simulink model "drive1m_real"  (R2022a)
settings: Solver=FixedStepAuto  StartTime=0.0  StopTime=10.0  RelTol=1e-3  EnableMultiTasking=on
values from neighbouring files (symbols this model uses):
  ticksPerRot = 20    [robotParameters.m]
  wheelR = 0.031    [robotParameters.m]
undefined symbols (not defined in the file or in its folder): InputPWM, WheelSpeed
libraries: arduinolib x8, slpidlib x1, mobileRoboticsTrainingLib x1
settings Model: ExtModeTrigDuration=2  Creator=heath  LastModifiedBy=heath
settings OptimizationCC: EnhancedBackFolding=on  PassReuseOutputArgsAs=Individual arguments  ZeroExternalMemoryAtStartup=off  ZeroInternalMemoryAtStartup=off  MaxStackSize=64  OptimizeBlockOrder=speed  DifferentSizesBufferReuse=on  OptimizationCustomize=off  EfficientTunableParamExpr=on
settings DebuggingCC: ParameterTunabilityLossMsg=error
settings HardwareCC: ProdBitPerPointer=32  ProdBitPerSizeT=32  ProdBitPerPtrDiffT=32  ProdLargestAtomicInteger=Long  ProdLargestAtomicFloat=Double  ProdWordSize=32  ProdHWDeviceType=ARM Compatible->ARM Cortex  UseEmbeddedCoderFeatures=off  UseSimulinkCoderFeatures=off
settings SFSimCC: MATLABDynamicMemAlloc=off
settings RTWCC: SystemTargetFile=ert.tlc  HardwareBoard=Arduino Nano 33 IoT  TemplateMakefile=ert_default_tmf  Toolchain=Arduino ARM  BuildConfiguration=Faster Runs
settings CodeAppCC: ForceParamTrailComments=on  IgnoreCustomStorageClasses=off  OperatorAnnotations=on  SimulinkDataObjDesc=on  SFDataObjDesc=on  InsertBlockDesc=on
settings ERTTargetCC: SupportContinuousTime=on  SupportNonInlinedSFcns=on  SupportVariableSizeSignals=on  ExtModeTransport=3  ExtModeStaticAlloc=on  ExtModeStaticAllocSize=8192  ExtModeMexFile=ext_xcp  ExtModeIntrfLevel=Level2 - Open

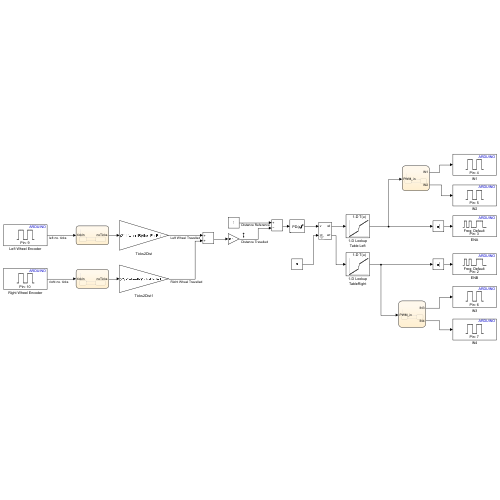
[thumbnail: Simulink's stored preview of the top-level diagram]
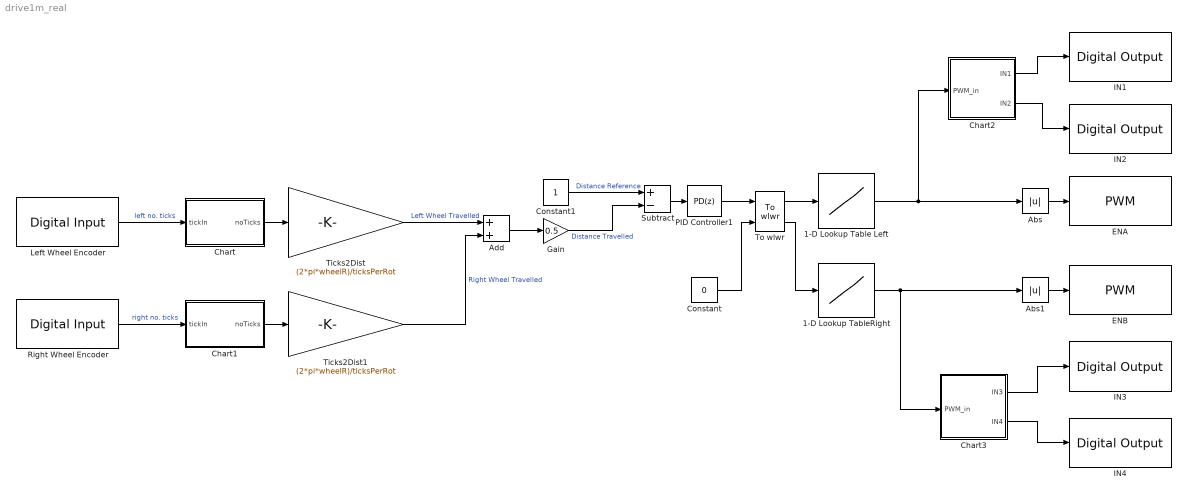
== system drive1m_real ==
  1-D Lookup Table Left : Lookup_n-D  NumberOfTableDimensions=1  BreakpointsForDimension1=WheelSpeed  Table=InputPWM  InternalRulePriority=Speed  RndMeth=Simplest
  1-D Lookup TableRight : Lookup_n-D  NumberOfTableDimensions=1  BreakpointsForDimension1=WheelSpeed  Table=InputPWM  InternalRulePriority=Speed  RndMeth=Simplest
  Abs : Abs  SaturateOnIntegerOverflow=off
  Abs1 : Abs  SaturateOnIntegerOverflow=off
  Add : Sum
  Chart : Stateflow chart  TreatAsAtomicUnit=on
  Chart1 : Stateflow chart  TreatAsAtomicUnit=on
  Chart2 : Stateflow chart  TreatAsAtomicUnit=on
  Chart3 : Stateflow chart  TreatAsAtomicUnit=on
  Constant : Constant  Value=0
  Constant1 : Constant
  ENA : arduinolib/PWM  pinNumber=3  frequencyType=Default  desiredFrequency=490.2  achievableFrequency=490.2
  ENB : arduinolib/PWM  pinNumber=2  frequencyType=Default  desiredFrequency=490.2  achievableFrequency=490.2
  Gain : Gain  Gain=0.5
  IN1 : arduinolib/Digital Output  pinNumber=4  Direction=output  blockPlatform=arduino
  IN2 : arduinolib/Digital Output  pinNumber=5  Direction=output  blockPlatform=arduino
  IN3 : arduinolib/Digital Output  pinNumber=6  Direction=output  blockPlatform=arduino
  IN4 : arduinolib/Digital Output  pinNumber=7  Direction=output  blockPlatform=arduino
  Left Wheel Encoder : arduinolib/Digital Input  pinNumber=9  mode=Default  Direction=input  SampleTime=0.1  blockPlatform=arduino
  PID Controller1 : slpidlib/PID Controller  Controller=PD  Form=Parallel  TimeDomain=Discrete-time  UseExternalTs=off  SampleTime=-1  IntegratorMethod=Forward Euler  FilterMethod=Forward Euler  ControllerParametersSource=internal  P=0.856187400165564  I=-30.3503190798584  UseKiTs=off  D=0.221941519902306  N=26.0006664672571  UseFilter=on  TunerSelectOption=Transfer Function Based (PID Tuner App)  InitialConditionSource=internal  InitialConditionForIntegrator=0  InitialConditionForFilter=0  DifferentiatorICPrevScaledInput=0  ExternalReset=none  TrackingMode=off  Kt=1  LimitOutput=on  SatLimitsSource=internal  UpperSaturationLimit=0.5  LowerSaturationLimit=-0.5  LinearizeAsGain=on  AntiWindupMode=clamping  Kb=1  POutMin=[]  POutMax=[]  IOutMin=[]  IOutMax=[]  DOutMin=[]  DOutMax=[]  NOutMin=[]  NOutMax=[]  SumOutMin=[]  SumOutMax=[]  SaturationOutMin=[]  SaturationOutMax=[]  PParamMin=[]  PParamMax=[]  IParamMin=[]  IParamMax=[]  DParamMin=[]  DParamMax=[]  NParamMin=[]  NParamMax=[]  KbParamMin=[]  KbParamMax=[]  KtParamMin=[]  KtParamMax=[]  KbOutMin=[]  KbOutMax=[]  KtOutMin=[]  KtOutMax=[]  IntegratorOutMin=[]  IntegratorOutMax=[]  FilterOutMin=[]  FilterOutMax=[]  SumI1OutMin=[]  SumI1OutMax=[]  SumI2OutMin=[]  SumI2OutMax=[]  SumI3OutMin=[]  SumI3OutMax=[]  SumI4OutMin=[]  SumI4OutMax=[]  SumDOutMin=[]  SumDOutMax=[]  DifferentiatorOutMin=[]  DifferentiatorOutMax=[]  FilterDiffOutCoefMin=[]  FilterDiffOutCoefMax=[]  ReciprocalOutMin=[]  ReciprocalOutMax=[]  SumDenOutMin=[]  SumDenOutMax=[]  SumNumOutMin=[]  SumNumOutMax=[]  DivideOutMin=[]  DivideOutMax=[]  UdiffTsProdOutMin=[]  UdiffTsProdOutMax=[]  NTsProdOutMin=[]  NTsProdOutMax=[]  UintegralTsProdOutMin=[]  UintegralTsProdOutMax=[]  UngainTsProdOutMin=[]  UngainTsProdOutMax=[]  IntegratorContinuousStateAttributes=''  IntegratorStateMustResolveToSignalObject=off  IntegratorRTWStateStorageClass=Auto  FilterContinuousStateAttributes=''  FilterStateMustResolveToSignalObject=off  FilterRTWStateStorageClass=Auto  ParallelPVariant=InternalParameters  IdealPVariant=Disabled  IVariant=Disabled  DVariant=InternalParameters  IntegratorVariant=Disabled  SatVariant=Enabled  AWVariant=Disabled  PCopyVariant=Disabled  TRVariant=Disabled  FdbkBlocksVariant=Forward  IdealPFdbkVariant=Disabled  SatFdbkVariant=Disabled  DerivativeFilterVariant=ForwardEulerFilter  NVariant=InternalParameters  NCopyVariant=Disabled  FilterICVariant=InternalICsFilter  IntegratorICVariant=Disabled  ExternalResetVariant=Disabled  TRSumVariant=Passthrough  SumFdbkVariant=Disabled  SumVariant=Sum_PD  TsampFilterVariant=InternalTs  TsampNgainVariant=Passthrough  TsampIntegralVariant=Disabled_SignalSpec  ExternalSaturationOutDataTypeStr=Inherit: Same as second input  aMode=0
  Right Wheel Encoder : arduinolib/Digital Input  pinNumber=10  mode=Default  Direction=input  SampleTime=0.1  blockPlatform=arduino
  Subtract : Sum  Inputs=+-
  Ticks2Dist : Gain  Gain=(2*pi*wheelR)/ticksPerRot
  Ticks2Dist1 : Gain  Gain=(2*pi*wheelR)/ticksPerRot
  To wlwr : mobileRoboticsTrainingLib/To wlwr  axleLength=axleLength  wheelR=wheelR
  wires:
  PID Controller1/1 -> To wlwr/1
  To wlwr/1 -> 1-D Lookup Table Left/1
  To wlwr/2 -> 1-D Lookup TableRight/1
  1-D Lookup TableRight/1 -> Chart3/1(PWM_in), Abs1/1
  Constant1/1 -> Subtract/1  "Distance Reference"
  Ticks2Dist/1 -> Add/1  "Left Wheel Travelled"
  1-D Lookup Table Left/1 -> Chart2/1(PWM_in), Abs/1
  Constant/1 -> To wlwr/2
  Gain/1 -> Subtract/2  "Distance Travelled"
  Subtract/1 -> PID Controller1/1
  Ticks2Dist1/1 -> Add/2  "Right Wheel Travelled"
  Add/1 -> Gain/1
  Left Wheel Encoder/1 -> Chart/1(tickIn)  "left no. ticks"
  Chart/1(noTicks) -> Ticks2Dist/1
  Right Wheel Encoder/1 -> Chart1/1(tickIn)  "right no. ticks"
  Chart1/1(noTicks) -> Ticks2Dist1/1
  Abs/1 -> ENA/1
  Abs1/1 -> ENB/1
  Chart2/1(IN1) -> IN1/1
  Chart2/2(IN2) -> IN2/1
  Chart3/1(IN3) -> IN3/1
  Chart3/2(IN4) -> IN4/1

== stateflow chart drive1m_real/Chart1 ==
  state NoTick
  state Tick
    entry:
    noTicks = noTicks + 1;
  (default) -> NoTick : {noTicks = 0;}
  Tick -> NoTick : [tickIn == 0]
  NoTick -> Tick : [tickIn == 1]
  data: noTicks output; tickIn input

== stateflow chart drive1m_real/Chart2 ==
  state Forward
    entry:
    IN1 = 1;
    IN2 = 0;
  state Back
    entry:
    IN1 = 0;
    IN2 = 1;
  (default) -> Forward
  Forward -> Back : [PWM_in<0]
  Back -> Forward : [PWM_in>=0]
  data: PWM_in input; IN1 output; IN2 output

== stateflow chart drive1m_real/Chart ==
  state NoTick
  state Tick
    entry:
    noTicks = noTicks + 1;
  (default) -> NoTick : {noTicks = 0;}
  Tick -> NoTick : [tickIn == 0]
  NoTick -> Tick : [tickIn == 1]
  data: noTicks output; tickIn input

== stateflow chart drive1m_real/Chart3 ==
  state Forward
    entry:
    IN4 = 1;
    IN3 = 0;
  state Back
    entry:
    IN4 = 0;
    IN3 = 1;
  (default) -> Forward
  Forward -> Back : [PWM_in<0]
  Back -> Forward : [PWM_in>=0]
  data: PWM_in input; IN3 output; IN4 output
